simulink model "State_Machine_Harness_DV"  (R2019b)
settings: Solver=FixedStepDiscrete  StartTime=0  StopTime=1.4000000000000001  FixedStep=0.10000000000000001  RelTol=1e-3  EnableMultiTasking=on
undefined symbols (not defined in the file): sigbuilder_block
settings Model: DataDictionary=DD_State_Machine.sldd  EnableAccessToBaseWorkspace=off  ExtModeTrigDuration=5  Creator=mdalbard  LastModifiedBy=cpatel
settings SolverCC: AutoInsertRateTranBlk=on
settings DataIOCC: ExternalInput=Battery  SaveOutput=off  SaveTime=off  SignalLoggingName=logsOut
settings OptimizationCC: BlockReduction=off  DefaultParameterBehavior=Inlined  UseDivisionForNetSlopeComputation=on  UseFloatMulNetSlope=on  DefaultUnderspecifiedDataType=single  UseSpecifiedMinMax=on  InlineInvariantSignals=on  ExpressionFolding=off  PassReuseOutputArgsAs=Individual arguments  ZeroExternalMemoryAtStartup=off  ZeroInternalMemoryAtStartup=off  NoFixptDivByZeroProtection=on  EfficientFloat2IntCast=on  LifeSpan=inf  MaxStackSize=64  OptimizeBlockOrder=speed  DifferentSizesBufferReuse=on  EfficientTunableParamExpr=on
settings DebuggingCC: SignalInfNanChecking=error  SaveWithParameterizedLinksMsg=none  UnderspecifiedInitializationDetection=Classic  MergeDetectMultiDrivingBlocksExec=none  CheckExecutionContextPreStartOutputMsg=on  CheckExecutionContextRuntimeOutputMsg=on  InheritedTsInSrcMsg=none  IntegerOverflowMsg=error  ParameterPrecisionLossMsg=none  ParameterTunabilityLossMsg=error  AssertControl=DisableAll  PregeneratedLibrarySubsystemCodeDiagnostic=none  SFUnexpectedBacktrackingDiag=warning  SFNoUnconditionalDefaultTransitionDiag=warning  SFExecutionAtInitializationDiag=none  ArithmeticOperatorsInVariantConditions=warning
settings HardwareCC: ProdBitPerPointer=32  ProdBitPerSizeT=32  ProdBitPerPtrDiffT=32  ProdLargestAtomicInteger=Long  ProdLargestAtomicFloat=Double  ProdEndianess=BigEndian  ProdWordSize=32  ProdLongLongMode=on  ProdHWDeviceType=Texas Instruments->TMS570 Cortex-R4
settings ModelReferenceCC: ModelReferenceNumInstancesAllowed=Single  PropagateSignalLabelsOutOfModel=off
settings SFSimCC: SimUseLocalCustomCode=off  MATLABDynamicMemAlloc=off  CustomCodeUndefinedFunction=UseInterfaceOnly
settings RTWCC: SystemTargetFile=ert.tlc  GenCodeOnly=on  TemplateMakefile=ert_default_tmf  GenerateReport=on  RTWUseLocalCustomCode=off  IncludeHyperlinkInReport=on  LaunchReport=on  GenerateTraceInfo=on  GenerateTraceReport=on  GenerateTraceReportSl=on  GenerateTraceReportSf=on  GenerateTraceReportEml=on  GenerateWebview=on  GenerateCodeMetricsReport=on
settings CodeAppCC: ForceParamTrailComments=on  IgnoreCustomStorageClasses=off  MaxIdLength=51  OperatorAnnotations=on  SimulinkDataObjDesc=on  SFDataObjDesc=on  MangleLength=4  InsertBlockDesc=on  ReqsInCode=on
settings ERTTargetCC: UtilityFuncGeneration=Shared location  GenerateSampleERTMain=on  IncludeMdlTerminateFcn=off  CombineSignalStateStructs=on  SuppressErrorStatus=on  SupportNonFinite=off  SupportComplex=off  ParenthesesLevel=Maximum  CastingMode=Standards  GenerateSharedConstants=off  InlinedParameterPlacement=NonHierarchical  ERTCustomFileTemplate=example_file_process.tlc  PreserveExpressionOrder=on  PreserveIfCondition=on  EnableSignedLeftShifts=off  EnableSignedRightShifts=off
settings ConfigComp: CovEnable=on  CovScope=ReferencedModels  CovIncludeTopModel=off  CovMetricSettings=dcmoe  CovHTMLOptions=-aTS=1 -bRG=1 -bTC=0 -hTR=0 -nFC=0 -scm=1 -bcm=1  CovHtmlReporting=on  CovSaveCumulativeToWorkspaceVar=on  CovSaveSingleToWorkspaceVar=on  CovModelRefEnable=on  DVMode=DesignErrorDetection  DVTestSuiteOptimization=Auto  DVDetectIntegerOverflow=off  DVRebuildModelRepresentation=Always

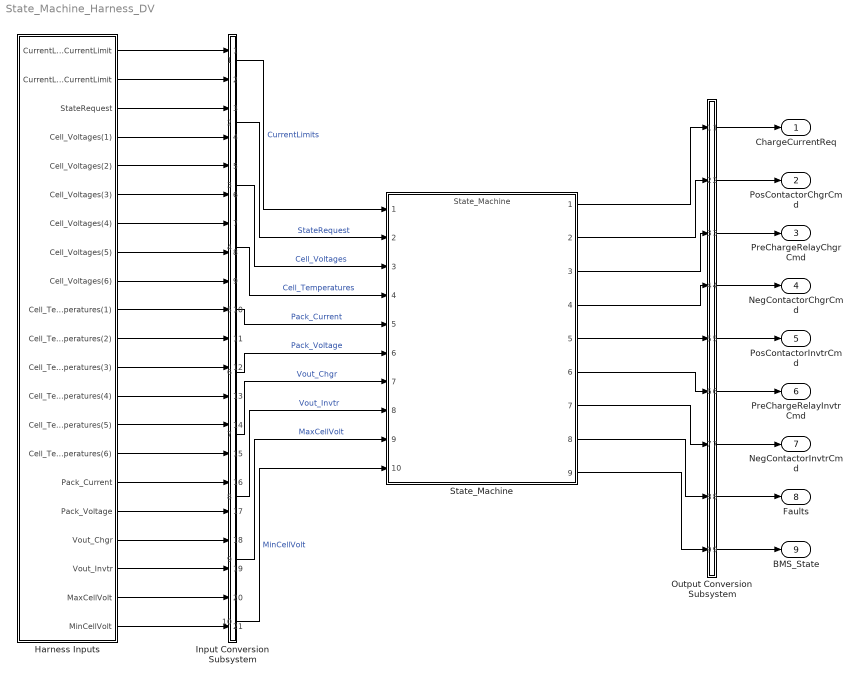
== system State_Machine_Harness_DV ==
  Harness Inputs : Subsystem  Tag=STV Subsys  LoadFcn=sigbuilder_block('load');  StartFcn=sigbuilder_block('start');  StopFcn=sigbuilder_block('stop');  ClipboardFcn=sigbuilder_block('clipboard');  mask(Sigbuilder block){tuvar=[0:10]}
      mask init:
      | if ~strcmp(get_param(bdroot(gcb),'SimulationStatus'),'stopped'),tuvar = sigbuilder_block('maskInit'); end
      settings: CopyFcn=sigbuilder_block('copy');  DeleteFcn=sigbuilder_block('delete');  ModelCloseFcn=sigbuilder_block('modelClose');  PreSaveFcn=sigbuilder_block('preSave');  PauseFcn=sigbuilder_block('pause');  ContinueFcn=sigbuilder_block('continue');  NameChangeFcn=sigbuilder_block('namechange');  OpenFcn=sigbuilder_block('open',[50 50 520 400 ]);  CloseFcn=sigbuilder_block('close');
      mask Display: plot(0, 0, 100, 100,[2, 2, 32, 32, 2], [68, 8, 8, 68, 68],[32, 2], [38, 38], [32, 19, 2],[53, 60, 44], [32, 17, 17, 2],[16, 16, 31, 31]);txt = getActiveGroup(gcbh);text(2, 100, txt,'verticalAlignment', 'top');
  Input Conversion Subsystem : Subsystem  Tag=__SLT_ICS__  Description=|
      | Signal spec.
      | and routing
      settings: AttributesFormatString=%<Description>
  Output Conversion Subsystem : Subsystem  Tag=__SLT_OCS__  Description=|
      | Signal spec.
      | and routing
      settings: AttributesFormatString=%<Description>
  State_Machine : ModelReference  ModelNameDialog=State_Machine  SimulationMode=Normal  ModelReferenceVersion=1.639
  ChargeCurrentReq : Outport  OutDataTypeStr=single  PortDimensions=[1]  VectorParamsAs1DForOutWhenUnconnected=off
  PosContactorChgrCmd : Outport  Port=2  OutDataTypeStr=boolean  PortDimensions=[1]  VectorParamsAs1DForOutWhenUnconnected=off
  PreChargeRelayChgrCmd : Outport  Port=3  OutDataTypeStr=boolean  PortDimensions=[1]  VectorParamsAs1DForOutWhenUnconnected=off
  NegContactorChgrCmd : Outport  Port=4  OutDataTypeStr=boolean  PortDimensions=[1]  VectorParamsAs1DForOutWhenUnconnected=off
  PosContactorInvtrCmd : Outport  Port=5  OutDataTypeStr=boolean  PortDimensions=[1]  VectorParamsAs1DForOutWhenUnconnected=off
  PreChargeRelayInvtrCmd : Outport  Port=6  OutDataTypeStr=boolean  PortDimensions=[1]  VectorParamsAs1DForOutWhenUnconnected=off
  NegContactorInvtrCmd : Outport  Port=7  OutDataTypeStr=boolean  PortDimensions=[1]  VectorParamsAs1DForOutWhenUnconnected=off
  Faults : Outport  Port=8  OutDataTypeStr=Bus: Faults  PortDimensions=1  VectorParamsAs1DForOutWhenUnconnected=off
  BMS_State : Outport  Port=9  OutDataTypeStr=Enum: BMS_State_Enum  PortDimensions=[1]  VectorParamsAs1DForOutWhenUnconnected=off
  wires:
  Harness Inputs/1(CurrentLimits.DischargeCurrentLimit) -> Input Conversion Subsystem/1(Inport_1)
  Harness Inputs/2(CurrentLimits.ChargeCurrentLimit) -> Input Conversion Subsystem/2(Inport_2)
  Harness Inputs/3(StateRequest) -> Input Conversion Subsystem/3(Inport_3)
  Harness Inputs/4(Cell_Voltages(1)) -> Input Conversion Subsystem/4(Inport_4)
  Harness Inputs/5(Cell_Voltages(2)) -> Input Conversion Subsystem/5(Inport_5)
  Harness Inputs/6(Cell_Voltages(3)) -> Input Conversion Subsystem/6(Inport_6)
  Harness Inputs/7(Cell_Voltages(4)) -> Input Conversion Subsystem/7(Inport_7)
  Harness Inputs/8(Cell_Voltages(5)) -> Input Conversion Subsystem/8(Inport_8)
  Harness Inputs/9(Cell_Voltages(6)) -> Input Conversion Subsystem/9(Inport_9)
  Harness Inputs/10(Cell_Temperatures(1)) -> Input Conversion Subsystem/10(Inport_10)
  Harness Inputs/11(Cell_Temperatures(2)) -> Input Conversion Subsystem/11(Inport_11)
  Harness Inputs/12(Cell_Temperatures(3)) -> Input Conversion Subsystem/12(Inport_12)
  Harness Inputs/13(Cell_Temperatures(4)) -> Input Conversion Subsystem/13(Inport_13)
  Harness Inputs/14(Cell_Temperatures(5)) -> Input Conversion Subsystem/14(Inport_14)
  Harness Inputs/15(Cell_Temperatures(6)) -> Input Conversion Subsystem/15(Inport_15)
  Harness Inputs/16(Pack_Current) -> Input Conversion Subsystem/16(Inport_16)
  Harness Inputs/17(Pack_Voltage) -> Input Conversion Subsystem/17(Inport_17)
  Harness Inputs/18(Vout_Chgr) -> Input Conversion Subsystem/18(Inport_18)
  Harness Inputs/19(Vout_Invtr) -> Input Conversion Subsystem/19(Inport_19)
  Harness Inputs/20(MaxCellVolt) -> Input Conversion Subsystem/20(Inport_20)
  Harness Inputs/21(MinCellVolt) -> Input Conversion Subsystem/21(Inport_21)
  Output Conversion Subsystem/1(Outport_1) -> ChargeCurrentReq/1
  Output Conversion Subsystem/2(Outport_2) -> PosContactorChgrCmd/1
  Output Conversion Subsystem/3(Outport_3) -> PreChargeRelayChgrCmd/1
  Output Conversion Subsystem/4(Outport_4) -> NegContactorChgrCmd/1
  Output Conversion Subsystem/5(Outport_5) -> PosContactorInvtrCmd/1
  Output Conversion Subsystem/6(Outport_6) -> PreChargeRelayInvtrCmd/1
  Output Conversion Subsystem/7(Outport_7) -> NegContactorInvtrCmd/1
  Output Conversion Subsystem/8(Outport_8) -> Faults/1
  Output Conversion Subsystem/9(Outport_9) -> BMS_State/1
  Input Conversion Subsystem/1(Outport_1) -> State_Machine/1  "CurrentLimits"
  Input Conversion Subsystem/2(Outport_2) -> State_Machine/2  "StateRequest"
  Input Conversion Subsystem/3(Outport_3) -> State_Machine/3  "Cell_Voltages"
  Input Conversion Subsystem/4(Outport_4) -> State_Machine/4  "Cell_Temperatures"
  Input Conversion Subsystem/5(Outport_5) -> State_Machine/5  "Pack_Current"
  Input Conversion Subsystem/6(Outport_6) -> State_Machine/6  "Pack_Voltage"
  Input Conversion Subsystem/7(Outport_7) -> State_Machine/7  "Vout_Chgr"
  Input Conversion Subsystem/8(Outport_8) -> State_Machine/8  "Vout_Invtr"
  Input Conversion Subsystem/9(Outport_9) -> State_Machine/9  "MaxCellVolt"
  Input Conversion Subsystem/10(Outport_10) -> State_Machine/10  "MinCellVolt"
  State_Machine/1 -> Output Conversion Subsystem/1(Inport_1)
  State_Machine/2 -> Output Conversion Subsystem/2(Inport_2)
  State_Machine/3 -> Output Conversion Subsystem/3(Inport_3)
  State_Machine/4 -> Output Conversion Subsystem/4(Inport_4)
  State_Machine/5 -> Output Conversion Subsystem/5(Inport_5)
  State_Machine/6 -> Output Conversion Subsystem/6(Inport_6)
  State_Machine/7 -> Output Conversion Subsystem/7(Inport_7)
  State_Machine/8 -> Output Conversion Subsystem/8(Inport_8)
  State_Machine/9 -> Output Conversion Subsystem/9(Inport_9)

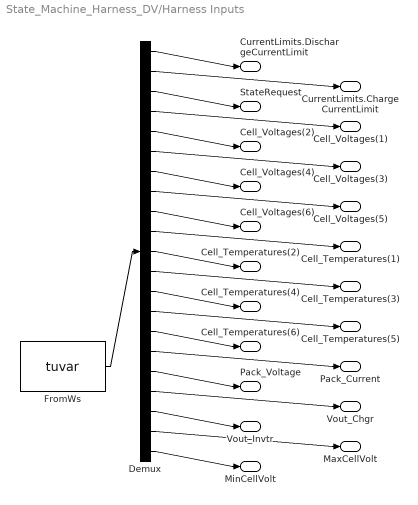
== system State_Machine_Harness_DV/Harness Inputs ==
  Demux : Demux  Tag=STV Demux  Outputs=21
  FromWs : FromWorkspace  Tag=STV FromWs  VariableName=tuvar  SampleTime=0
  CurrentLimits.DischargeCurrentLimit : Outport  Tag=STV Outport  VectorParamsAs1DForOutWhenUnconnected=off
  CurrentLimits.ChargeCurrentLimit : Outport  Tag=STV Outport  Port=2  VectorParamsAs1DForOutWhenUnconnected=off
  StateRequest : Outport  Tag=STV Outport  Port=3  VectorParamsAs1DForOutWhenUnconnected=off
  Cell_Voltages(1) : Outport  Tag=STV Outport  Port=4  VectorParamsAs1DForOutWhenUnconnected=off
  Cell_Voltages(2) : Outport  Tag=STV Outport  Port=5  VectorParamsAs1DForOutWhenUnconnected=off
  Cell_Voltages(3) : Outport  Tag=STV Outport  Port=6  VectorParamsAs1DForOutWhenUnconnected=off
  Cell_Voltages(4) : Outport  Tag=STV Outport  Port=7  VectorParamsAs1DForOutWhenUnconnected=off
  Cell_Voltages(5) : Outport  Tag=STV Outport  Port=8  VectorParamsAs1DForOutWhenUnconnected=off
  Cell_Voltages(6) : Outport  Tag=STV Outport  Port=9  VectorParamsAs1DForOutWhenUnconnected=off
  Cell_Temperatures(1) : Outport  Tag=STV Outport  Port=10  VectorParamsAs1DForOutWhenUnconnected=off
  Cell_Temperatures(2) : Outport  Tag=STV Outport  Port=11  VectorParamsAs1DForOutWhenUnconnected=off
  Cell_Temperatures(3) : Outport  Tag=STV Outport  Port=12  VectorParamsAs1DForOutWhenUnconnected=off
  Cell_Temperatures(4) : Outport  Tag=STV Outport  Port=13  VectorParamsAs1DForOutWhenUnconnected=off
  Cell_Temperatures(5) : Outport  Tag=STV Outport  Port=14  VectorParamsAs1DForOutWhenUnconnected=off
  Cell_Temperatures(6) : Outport  Tag=STV Outport  Port=15  VectorParamsAs1DForOutWhenUnconnected=off
  Pack_Current : Outport  Tag=STV Outport  Port=16  VectorParamsAs1DForOutWhenUnconnected=off
  Pack_Voltage : Outport  Tag=STV Outport  Port=17  VectorParamsAs1DForOutWhenUnconnected=off
  Vout_Chgr : Outport  Tag=STV Outport  Port=18  VectorParamsAs1DForOutWhenUnconnected=off
  Vout_Invtr : Outport  Tag=STV Outport  Port=19  VectorParamsAs1DForOutWhenUnconnected=off
  MaxCellVolt : Outport  Tag=STV Outport  Port=20  VectorParamsAs1DForOutWhenUnconnected=off
  MinCellVolt : Outport  Tag=STV Outport  Port=21  VectorParamsAs1DForOutWhenUnconnected=off
  wires:
  FromWs/1 -> Demux/1
  Demux/1 -> CurrentLimits.DischargeCurrentLimit/1
  Demux/2 -> CurrentLimits.ChargeCurrentLimit/1
  Demux/3 -> StateRequest/1
  Demux/4 -> Cell_Voltages(1)/1
  Demux/5 -> Cell_Voltages(2)/1
  Demux/6 -> Cell_Voltages(3)/1
  Demux/7 -> Cell_Voltages(4)/1
  Demux/8 -> Cell_Voltages(5)/1
  Demux/9 -> Cell_Voltages(6)/1
  Demux/10 -> Cell_Temperatures(1)/1
  Demux/11 -> Cell_Temperatures(2)/1
  Demux/12 -> Cell_Temperatures(3)/1
  Demux/13 -> Cell_Temperatures(4)/1
  Demux/14 -> Cell_Temperatures(5)/1
  Demux/15 -> Cell_Temperatures(6)/1
  Demux/16 -> Pack_Current/1
  Demux/17 -> Pack_Voltage/1
  Demux/18 -> Vout_Chgr/1
  Demux/19 -> Vout_Invtr/1
  Demux/20 -> MaxCellVolt/1
  Demux/21 -> MinCellVolt/1

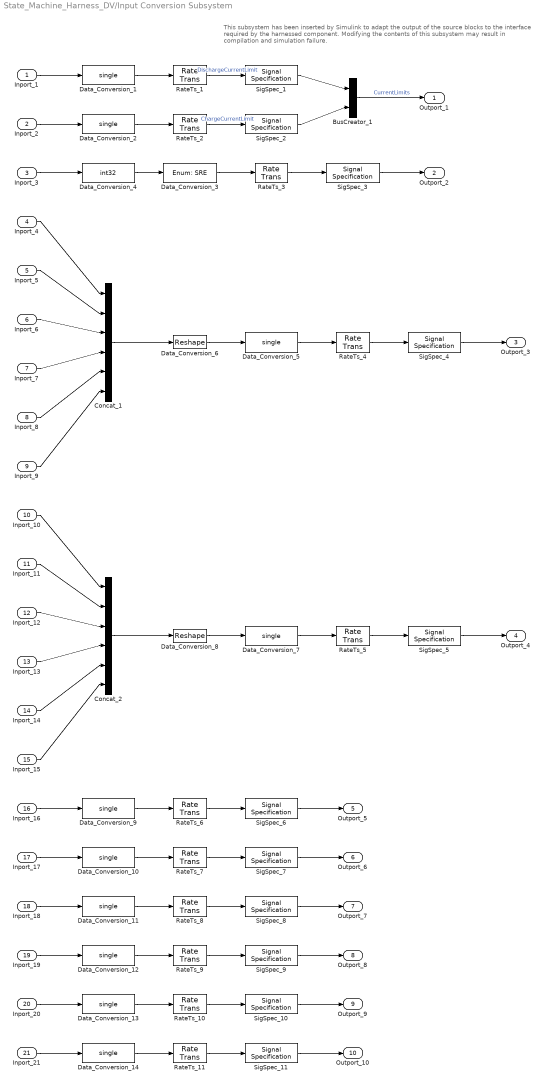
== system State_Machine_Harness_DV/Input Conversion Subsystem ==
  note: This subsystem has been inserted by Simulink to adapt the output of the source blocks to the interface required by the harnessed component.
      |  Modifying the contents of this subsystem may result in compilation and simulation failure.
  Inport_1 : Inport
  Inport_2 : Inport  Port=2
  Inport_3 : Inport  Port=3
  Inport_4 : Inport  Port=4
  Inport_5 : Inport  Port=5
  Inport_6 : Inport  Port=6
  Inport_7 : Inport  Port=7
  Inport_8 : Inport  Port=8
  Inport_9 : Inport  Port=9
  Inport_10 : Inport  Port=10
  Inport_11 : Inport  Port=11
  Inport_12 : Inport  Port=12
  Inport_13 : Inport  Port=13
  Inport_14 : Inport  Port=14
  Inport_15 : Inport  Port=15
  Inport_16 : Inport  Port=16
  Inport_17 : Inport  Port=17
  Inport_18 : Inport  Port=18
  Inport_19 : Inport  Port=19
  Inport_20 : Inport  Port=20
  Inport_21 : Inport  Port=21
  BusCreator_1 : BusCreator  Inputs=2  OutDataTypeStr=Bus: CurrentLimits
  Concat_1 : Concatenate  NumInputs=6
  Concat_2 : Concatenate  NumInputs=6
  Data_Conversion_{1..2,5,7,9..14} (10 alike) : DataTypeConversion  OutDataTypeStr=single  SaturateOnIntegerOverflow=on  RndMeth=Zero
  Data_Conversion_3 : DataTypeConversion  OutDataTypeStr=Enum: SRE  SaturateOnIntegerOverflow=on  RndMeth=Zero
  Data_Conversion_4 : DataTypeConversion  OutDataTypeStr=int32  RndMeth=Round  SaturateOnIntegerOverflow=on
  Data_Conversion_6 : Reshape  OutputDimensionality=Customize  OutputDimensions=[6]
  Data_Conversion_8 : Reshape  OutputDimensionality=Customize  OutputDimensions=[6]
  RateTs_{1..11} (11 alike) : RateTransition  OutPortSampleTime=0.1
  SigSpec_{1..2,6..11} (8 alike) : SignalSpecification  OutDataTypeStr=single  Dimensions=[1]  SampleTime=0.1
  SigSpec_3 : SignalSpecification  OutDataTypeStr=Enum: SRE  Dimensions=[1]  SampleTime=0.1
  SigSpec_4 : SignalSpecification  OutDataTypeStr=single  Dimensions=[6]  SampleTime=0.1
  SigSpec_5 : SignalSpecification  OutDataTypeStr=single  Dimensions=[6]  SampleTime=0.1
  Outport_1 : Outport  VectorParamsAs1DForOutWhenUnconnected=off
  Outport_2 : Outport  Port=2  VectorParamsAs1DForOutWhenUnconnected=off
  Outport_3 : Outport  Port=3  VectorParamsAs1DForOutWhenUnconnected=off
  Outport_4 : Outport  Port=4  VectorParamsAs1DForOutWhenUnconnected=off
  Outport_5 : Outport  Port=5  VectorParamsAs1DForOutWhenUnconnected=off
  Outport_6 : Outport  Port=6  VectorParamsAs1DForOutWhenUnconnected=off
  Outport_7 : Outport  Port=7  VectorParamsAs1DForOutWhenUnconnected=off
  Outport_8 : Outport  Port=8  VectorParamsAs1DForOutWhenUnconnected=off
  Outport_9 : Outport  Port=9  VectorParamsAs1DForOutWhenUnconnected=off
  Outport_10 : Outport  Port=10  VectorParamsAs1DForOutWhenUnconnected=off
  wires:
  BusCreator_1/1 -> Outport_1/1  "CurrentLimits"
  SigSpec_1/1 -> BusCreator_1/1
  RateTs_1/1 -> SigSpec_1/1  "DischargeCurrentLimit"
  Data_Conversion_1/1 -> RateTs_1/1
  Inport_1/1 -> Data_Conversion_1/1
  SigSpec_2/1 -> BusCreator_1/2
  RateTs_2/1 -> SigSpec_2/1  "ChargeCurrentLimit"
  Data_Conversion_2/1 -> RateTs_2/1
  Inport_2/1 -> Data_Conversion_2/1
  SigSpec_3/1 -> Outport_2/1
  RateTs_3/1 -> SigSpec_3/1
  Data_Conversion_3/1 -> RateTs_3/1
  Data_Conversion_4/1 -> Data_Conversion_3/1
  Inport_3/1 -> Data_Conversion_4/1
  SigSpec_4/1 -> Outport_3/1
  RateTs_4/1 -> SigSpec_4/1
  Data_Conversion_5/1 -> RateTs_4/1
  Data_Conversion_6/1 -> Data_Conversion_5/1
  Concat_1/1 -> Data_Conversion_6/1
  Inport_4/1 -> Concat_1/1
  Inport_5/1 -> Concat_1/2
  Inport_6/1 -> Concat_1/3
  Inport_7/1 -> Concat_1/4
  Inport_8/1 -> Concat_1/5
  Inport_9/1 -> Concat_1/6
  SigSpec_5/1 -> Outport_4/1
  RateTs_5/1 -> SigSpec_5/1
  Data_Conversion_7/1 -> RateTs_5/1
  Data_Conversion_8/1 -> Data_Conversion_7/1
  Concat_2/1 -> Data_Conversion_8/1
  Inport_10/1 -> Concat_2/1
  Inport_11/1 -> Concat_2/2
  Inport_12/1 -> Concat_2/3
  Inport_13/1 -> Concat_2/4
  Inport_14/1 -> Concat_2/5
  Inport_15/1 -> Concat_2/6
  SigSpec_6/1 -> Outport_5/1
  RateTs_6/1 -> SigSpec_6/1
  Data_Conversion_9/1 -> RateTs_6/1
  Inport_16/1 -> Data_Conversion_9/1
  SigSpec_7/1 -> Outport_6/1
  RateTs_7/1 -> SigSpec_7/1
  Data_Conversion_10/1 -> RateTs_7/1
  Inport_17/1 -> Data_Conversion_10/1
  SigSpec_8/1 -> Outport_7/1
  RateTs_8/1 -> SigSpec_8/1
  Data_Conversion_11/1 -> RateTs_8/1
  Inport_18/1 -> Data_Conversion_11/1
  SigSpec_9/1 -> Outport_8/1
  RateTs_9/1 -> SigSpec_9/1
  Data_Conversion_12/1 -> RateTs_9/1
  Inport_19/1 -> Data_Conversion_12/1
  SigSpec_10/1 -> Outport_9/1
  RateTs_10/1 -> SigSpec_10/1
  Data_Conversion_13/1 -> RateTs_10/1
  Inport_20/1 -> Data_Conversion_13/1
  SigSpec_11/1 -> Outport_10/1
  RateTs_11/1 -> SigSpec_11/1
  Data_Conversion_14/1 -> RateTs_11/1
  Inport_21/1 -> Data_Conversion_14/1

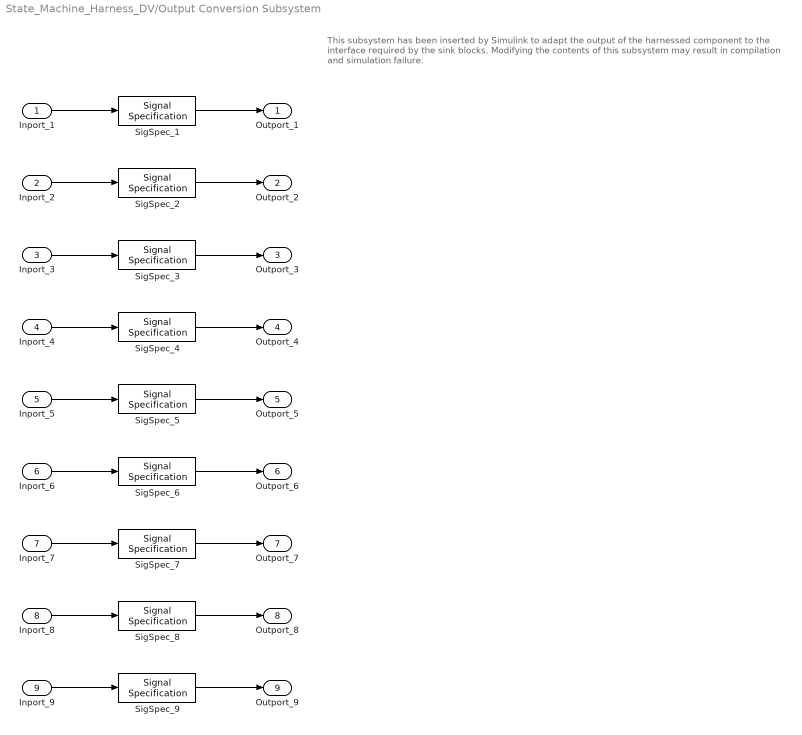
== system State_Machine_Harness_DV/Output Conversion Subsystem ==
  note: This subsystem has been inserted by Simulink to adapt the output of the harnessed component to the interface required by the sink blocks.
      |  Modifying the contents of this subsystem may result in compilation and simulation failure.
  Inport_1 : Inport
  Inport_2 : Inport  Port=2
  Inport_3 : Inport  Port=3
  Inport_4 : Inport  Port=4
  Inport_5 : Inport  Port=5
  Inport_6 : Inport  Port=6
  Inport_7 : Inport  Port=7
  Inport_8 : Inport  Port=8
  Inport_9 : Inport  Port=9
  SigSpec_1 : SignalSpecification  OutDataTypeStr=single  Dimensions=[1]  SampleTime=0.1
  SigSpec_{2..7} (6 alike) : SignalSpecification  OutDataTypeStr=boolean  Dimensions=[1]  SampleTime=0.1
  SigSpec_8 : SignalSpecification  OutDataTypeStr=Bus: Faults  Dimensions=[1]  SampleTime=0.1
  SigSpec_9 : SignalSpecification  OutDataTypeStr=Enum: BMS_State_Enum  Dimensions=[1]  SampleTime=0.1
  Outport_1 : Outport  VectorParamsAs1DForOutWhenUnconnected=off
  Outport_2 : Outport  Port=2  VectorParamsAs1DForOutWhenUnconnected=off
  Outport_3 : Outport  Port=3  VectorParamsAs1DForOutWhenUnconnected=off
  Outport_4 : Outport  Port=4  VectorParamsAs1DForOutWhenUnconnected=off
  Outport_5 : Outport  Port=5  VectorParamsAs1DForOutWhenUnconnected=off
  Outport_6 : Outport  Port=6  VectorParamsAs1DForOutWhenUnconnected=off
  Outport_7 : Outport  Port=7  VectorParamsAs1DForOutWhenUnconnected=off
  Outport_8 : Outport  Port=8  VectorParamsAs1DForOutWhenUnconnected=off
  Outport_9 : Outport  Port=9  VectorParamsAs1DForOutWhenUnconnected=off
  wires:
  Inport_1/1 -> SigSpec_1/1
  SigSpec_1/1 -> Outport_1/1
  Inport_2/1 -> SigSpec_2/1
  SigSpec_2/1 -> Outport_2/1
  Inport_3/1 -> SigSpec_3/1
  SigSpec_3/1 -> Outport_3/1
  Inport_4/1 -> SigSpec_4/1
  SigSpec_4/1 -> Outport_4/1
  Inport_5/1 -> SigSpec_5/1
  SigSpec_5/1 -> Outport_5/1
  Inport_6/1 -> SigSpec_6/1
  SigSpec_6/1 -> Outport_6/1
  Inport_7/1 -> SigSpec_7/1
  SigSpec_7/1 -> Outport_7/1
  Inport_8/1 -> SigSpec_8/1
  SigSpec_8/1 -> Outport_8/1
  Inport_9/1 -> SigSpec_9/1
  SigSpec_9/1 -> Outport_9/1
